simulink model "Motion_planner_Street_Drone"  (R2019b)
settings: Solver=FixedStepAuto  StartTime=0.0  StopTime=25  FixedStep=0.0075  MaxStep=1e-1  MinStep=1e-3  RelTol=1e-3  AbsTol=1e-4
InitFcn:
  | SD_init1
values from neighbouring files (symbols this model uses):
  cost = [2.71432892747 3.32441927977 3.79268757264 4.85642115368 6.12135035287 7.09825974303 9.57278659789 1.55754789407 1.51399555616 2.57723707661 3.8468529147 4.8336387623 ... (2430 elements, 1x2430)]    [matlab.mat]
  Front_brake = [0 2.2085352751 4.15209150797 6.12733711785 8.16604105928 9.79119154879 12.1808659635 14.1242630413 16.1155522836 18.1386900579 20.0839213981 22.1313006548 ... (68 elements, 34x2)]    [Front_brake.mat]
  N = size(X,1)    [curvature.m]
  obsx = [dx1 dx2 dx3 dx4]'    [dynamic_collison.m]    (also in dynamic_detection1.m = [x1 x2 x3 x4]')
  obsy = [dy1 dy2 dy3 dy4]'    [dynamic_collison.m]    (also in dynamic_detection1.m = [y1 y2 y3 y4]')
  x = obs_path(i,1)    [dynamic_collison.m]    (also in dynamic_detection1.m)
  X = [X]    [curvature.m]
  y = obs_path(i,2)    [dynamic_collison.m]    (also in dynamic_detection1.m)
undefined symbols (not defined in the file or in its folder): d, dfin, dini, Ki, Kp, L_0f, lookahead_time, lookahead_time_rev, Rear_brake, sigbuilder_block, steer_ratio, steer_sens, tfin, tini, TPS_0, xfin, Y, yfin, Z
libraries: sm_lib x290, nesl_utility x136, simulink x6, vrlib x2, powerlib_meascontrol x2
(part 2 of 14)

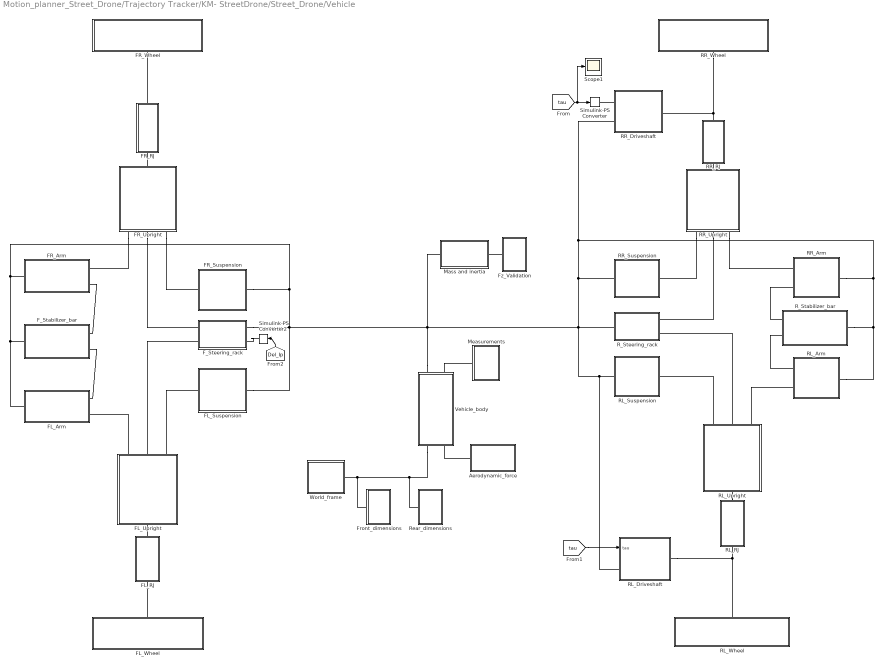
== system Motion_planner_Street_Drone/Trajectory Tracker/KM- StreetDrone/Street_Drone/Vehicle ==
  Aerodynamic_force : Subsystem
  FL_Arm : Subsystem
  FL_RJ : Subsystem
  FL_Suspension : Subsystem
  FL_Upright : Subsystem
  FL_Wheel : Subsystem
  FR_Arm : Subsystem
  FR_RJ : Subsystem
  FR_Suspension : Subsystem
  FR_Upright : Subsystem
  FR_Wheel : Subsystem
  F_Stabilizer_bar : Subsystem
  F_Steering_rack : Subsystem
  Front_dimensions : Subsystem
  Fz_Validation : Subsystem
  Mass and inertia : Subsystem
  Measurements : Subsystem
  RL_Arm : Subsystem
  RL_Driveshaft : Subsystem
  RL_RJ : Subsystem
  RL_Suspension : Subsystem
  RL_Upright : Subsystem
  RL_Wheel : Subsystem
  RR_Arm : Subsystem
  RR_Driveshaft : Subsystem
  RR_RJ : Subsystem
  RR_Suspension : Subsystem
  RR_Upright : Subsystem
  RR_Wheel : Subsystem
  R_Stabilizer_bar : Subsystem
  R_Steering_rack : Subsystem
  Rear_dimensions : Subsystem
  Scope1 : Scope
  Simulink-PS Converter : nesl_utility/Simulink-PS Converter  PhysicalDomain=network_engine_domain  SubClassName=ps_input  LeftPortType=input  RightPortType=output  PseudoPeriodic=off  Frequencies=[]  NoiseDistribution=none  NoiseParameters=[]  Unit=1  AffineConversion=off  FilteringAndDerivatives=provide  SimscapeFilterOrder=1  InputFilterTimeConstant=0.001  UdotUserProvided=0
  Simulink-PS Converter2 : nesl_utility/Simulink-PS Converter  PhysicalDomain=network_engine_domain  SubClassName=ps_input  LeftPortType=input  RightPortType=output  PseudoPeriodic=off  Frequencies=[]  NoiseDistribution=none  NoiseParameters=[]  Unit=cm  AffineConversion=off  FilteringAndDerivatives=filter  SimscapeFilterOrder=2  InputFilterTimeConstant=0.001  UdotUserProvided=0
  Vehicle_body : Subsystem
  World_frame : Subsystem
  wires:
  [tau] -> RL_Driveshaft/1(tau)
  [Del_Ip] -> Simulink-PS Converter2/1
  [tau] -> Simulink-PS Converter/1, Scope1/1
  connections:
  Fz_Validation/LConn1 -- Mass and inertia/RConn1
  RR_RJ/RConn1 -- RR_Wheel/LConn1 -- RR_Driveshaft/RConn1
  RL_RJ/RConn1 -- RL_Wheel/LConn1 -- RL_Driveshaft/RConn1
  FL_Wheel/LConn1 -- FL_RJ/RConn1
  FR_RJ/RConn1 -- FR_Wheel/LConn1
  FR_Arm/RConn2 -- F_Stabilizer_bar/RConn1
  Aerodynamic_force/LConn1 -- Vehicle_body/RConn2
  FR_Upright/LConn1 -- FR_Arm/RConn1
  RR_Upright/RConn1 -- RR_RJ/LConn1
  RR_Driveshaft/LConn1 -- Simulink-PS Converter/RConn1
  RL_Upright/LConn1 -- RL_RJ/LConn1
  Measurements/RConn1 -- Vehicle_body/LConn2
  World_frame/RConn1 -- Front_dimensions/LConn1 -- Rear_dimensions/LConn1 -- Vehicle_body/RConn1
  FL_Upright/RConn1 -- FL_RJ/LConn1
  RL_Upright/RConn1 -- RL_Suspension/RConn1
  RR_Upright/LConn1 -- RR_Suspension/RConn1
  FR_Upright/LConn2 -- F_Steering_rack/RConn1
  RR_Upright/LConn3 -- RR_Arm/RConn1
  FR_RJ/LConn1 -- FR_Upright/RConn1
  FL_Upright/LConn2 -- F_Steering_rack/RConn2
  RL_Upright/RConn3 -- RL_Arm/RConn2
  RR_Upright/LConn2 -- R_Steering_rack/RConn1
  Vehicle_body/LConn1 -- RR_Suspension/LConn1 -- RR_Arm/LConn1 -- RL_Arm/LConn1 -- R_Stabilizer_bar/LConn1 -- RR_Driveshaft/LConn2 -- R_Steering_rack/LConn1 -- RL_Suspension/LConn1 -- RL_Driveshaft/LConn1 -- Mass and inertia/LConn1 -- FL_Suspension/LConn1 -- F_Steering_rack/LConn1 -- FR_Suspension/LConn1 -- FR_Arm/LConn1 -- F_Stabilizer_bar/LConn1 -- FL_Arm/LConn1
  FR_Upright/LConn3 -- FR_Suspension/RConn1
  RL_Upright/RConn2 -- R_Steering_rack/RConn2
  R_Stabilizer_bar/RConn1 -- RR_Arm/RConn2
  Simulink-PS Converter2/RConn1 -- F_Steering_rack/LConn2
  FL_Upright/LConn1 -- FL_Arm/RConn2
  F_Stabilizer_bar/RConn2 -- FL_Arm/RConn1
  FL_Upright/LConn3 -- FL_Suspension/RConn1
  RL_Arm/RConn1 -- R_Stabilizer_bar/RConn2

== system Motion_planner_Street_Drone/Trajectory Tracker/KM- StreetDrone/Street_Drone/Inputs/Del ==
  del : Inport
  Constant2 : Constant  Value=0
  Del : Subsystem  Tag=STV Subsys  LoadFcn=sigbuilder_block('load');  StartFcn=sigbuilder_block('start');  StopFcn=sigbuilder_block('stop');  ClipboardFcn=sigbuilder_block('clipboard');  mask(Sigbuilder block){tuvar=[0:10]}
      mask help: Simulink:masks:SigbuilderBlock_MD
      mask init:
      | if ~strcmp(get_param(bdroot(gcbh),'SimulationStatus'),'stopped') tuvar = sigbuilder_block('maskInit'); end
      settings: CopyFcn=sigbuilder_block('copy');  DeleteFcn=sigbuilder_block('delete');  ModelCloseFcn=sigbuilder_block('modelClose');  PreSaveFcn=sigbuilder_block('preSave');  PauseFcn=sigbuilder_block('pause');  ContinueFcn=sigbuilder_block('continue');  NameChangeFcn=sigbuilder_block('namechange');  OpenFcn=sigbuilder_block('open',[5.4 72.6 1141.2 513.6 ]);  CloseFcn=sigbuilder_block('close');
      mask Display: plot(0, 0, 100, 100,[2, 2, 32, 32, 2], [68, 8, 8, 68, 68],[32, 2], [38, 38], [32, 19, 2],[53, 60, 44], [32, 17, 17, 2],[16, 16, 31, 31]);txt = getActiveGroup(gcbh);text(2, 100, txt,'verticalAlignment', 'top');
  Manual Switch1 : ManualSwitch
  Manual Switch3 : ManualSwitch  CurrentSetting=0
  Radius_of_pinion_cms : Gain  Gain=0.56
  Scope : Scope
  To Workspace : ToWorkspace  VariableName=del_hand_wheel  SampleTime=-1
  steering_ratio : Gain  Gain=14.0166
  to_degrees : Gain  Gain=180/pi
  to_radians : Gain  Gain=pi/180
  tag scope: Del_Ip=global, Del_Ip_hand=global
  wires:
  Del/1(Signal 1) -> Manual Switch1/2
  steering_ratio/1 -> Manual Switch1/1
  to_degrees/1 -> steering_ratio/1
  del/1 -> to_degrees/1
  Manual Switch3/1 -> Scope/1, [Del_Ip]
  Manual Switch1/1 -> To Workspace/1, [Del_Ip_hand], Radius_of_pinion_cms/1
  to_radians/1 -> Manual Switch3/2
  Radius_of_pinion_cms/1 -> to_radians/1
  Constant2/1 -> Manual Switch3/1

== system Motion_planner_Street_Drone/Trajectory Tracker/KM- StreetDrone/Street_Drone/Inputs/Velocity ==
  Vel : Inport
  Manual Switch2 : ManualSwitch  CurrentSetting=0
  Normal_manoever : Subsystem
  tag scope: Inputs=global
  wires:
  Vel/1 -> Manual Switch2/2
  Manual Switch2/1 -> [Inputs]
  Normal_manoever/1(Out1) -> Manual Switch2/1

== system Motion_planner_Street_Drone/Trajectory Tracker/KM- StreetDrone/Street_Drone/Powertrain and Brake System1/Brake_system ==
  I/p : Inport
  Brake_pedal : Saturate  UpperLimit=0  LowerLimit=-100
  Front_brake : Lookup_n-D  NumberOfTableDimensions=1  BreakpointsForDimension1=[Front_brake(:,1)]  Table=[Front_brake(:,2)]  InternalRulePriority=Speed  RndMeth=Simplest  InputSameDT=on
  Gain1 : Gain  Gain=-1
  Gain11 : Gain  Gain=-1/100
  Gain2 : Gain  Gain=0.5
  Gain3 : Gain  Gain=0.5
  Max_Br_pr : Gain  Gain=71.7
  Rear_brake : Lookup_n-D  NumberOfTableDimensions=1  BreakpointsForDimension1=[Rear_brake(:,1)]  Table=[Rear_brake(:,2)]  InternalRulePriority=Speed  RndMeth=Simplest  InputSameDT=on
  Scope{25,28..29,31} (4 alike) : Scope
  To Workspace1 : ToWorkspace  VariableName=brake_pr  SampleTime=-1
  To Workspace2 : ToWorkspace  VariableName=brake_pedal  SampleTime=-1
  tag scope: brTau_F=global, brTau_R=global, br_pedal=global
  wires:
  Gain3/1 -> [brTau_R]
  Gain2/1 -> [brTau_F]
  Max_Br_pr/1 -> Front_brake/1, To Workspace1/1, Scope31/1, Rear_brake/1
  Rear_brake/1 -> Scope28/1, Gain3/1
  Front_brake/1 -> Scope25/1, Gain2/1
  Gain11/1 -> Gain1/1, Max_Br_pr/1
  Brake_pedal/1 -> Scope29/1, Gain11/1
  I/p/1 -> Brake_pedal/1
  Gain1/1 -> To Workspace2/1, [br_pedal]

== system Motion_planner_Street_Drone/Trajectory Tracker/KM- StreetDrone/Street_Drone/Powertrain and Brake System1/Driveline_viscous_losses ==
  Gain : Gain  Gain=-1
  Product : Product
  Scope : Scope
  Scope1 : Scope
  Switch : Switch
  Viscous_friction1 : Gain  Commented=on  Gain=2
  Viscous_friction2 : Gain  Gain=2.537
  O/p : Outport
  tag scope: PT_loss=global
  wires:
  [motor_tau] -> Switch/2
  Gain/1 -> Switch/3
  Switch/1 -> O/p/1, Scope/1
  Product/1 -> Switch/1, Gain/1
  [RL_Re] -> Product/2
  Viscous_friction2/1 -> Product/1, Scope1/1, [PT_loss]
  [Vel] -> Viscous_friction2/1

== system Motion_planner_Street_Drone/Trajectory Tracker/KM- StreetDrone/Street_Drone/Powertrain and Brake System1/Motor ==
  I/p2 : Inport
  I/p1 : Inport  Port=2
  % : Gain  Gain=1/100
  %1 : Gain  Gain=100
  2-D Lookup Table2 : Lookup_n-D  BreakpointsForDimension1=[0 0.1 0.2 0.3 0.4 0.5 0.6 0.7 0.8 0.9 1]  BreakpointsForDimension2=[TPS_0(:,1)]  Table=[-90.24,-90.26,-90.24,-90.22,-90.23,-86.63,-72.71,-56.25,-50.21,-44.59,-40.69,-37.61,-34.44,-31.97,-29.79,-27.98,-26.37,-24.7,-23.15,-22.11,-21.24,-20.43,-19.47,-18.66,-17.94,-17.25,-16.58,-15.87,-15.16,-14.33,-14.11,-14.27,-14.21,-13.57,-12.89,-12.82,-12.72,-12.45,-12.19,-11.94,-11.65,-11.38,-10.97,-10.65;-25.48,-25.71,-26.16,-26.77,-27.52,-28.39,-29.45,-30.61,-30.61,-30.63,-30.66,-30.57,-29.83,-28.1,-26.6,-25.1,-23.88,-22.46,-21.12,-19.91,-18.49,-17.4,-16.44,-15.32,-14.29,-13.12,-11.74,-10.25,-9.37,-8.72,-8.56,-8.89,-9.14,-8.69,-8.35,-8.5,-8.76,-8.73,-8.69,-8.74,-8.78,-8.93,-8.85,-8.81;-3.28,-3.05,-2.62,-2.39,-2.44,-2.48,-2.54,-2.68,-2.6,-2.61,-2.62,-2.68,-2.68,-2.82,-2.75,-2.82,-2.8,-2.89,-2.94,-2.63,-2.34,-2.19,-2.46,-2.64,-2.54,-2.48,-2.51,-2.49,-2.26,-2.06,-2.09,-2.06,-2.16,-2.2,-2.19,-2.17,-2.12,-2.11,-2.09,-2.23,-2.18,-2.22,-1.91,-1.71;1.59,1.32,0.82,0.49,0.72,0.7,0.69,0.55,0.55,0.52,0.54,0.5,0.5,0.39,0.41,0.36,0.38,0.23,0.01,0.14,0.44,0.56,0.42,0.38,0.4,0.46,0.52,0.71,0.75,0.99,0.75,0.46,0.17,0.45,0.71,0.69,0.65,0.71,0.82,0.8,0.7,0.73,0.91,0.92;5.53,5.09,4.45,4.29,4.5,4.55,4.53,4.39,4.32,4.22,4.1,4.06,4.01,3.82,3.78,3.79,3.8,3.5,3.19,3.26,3.52,3.61,3.6,3.59,3.55,3.57,3.62,3.78,3.97,3.97,3.63,3.07,2.54,3,3.46,3.3,3.14,3.1,3.27,3.29,3.3,3.06,2.88,2.84;11.33,11.26,11.2,11.21,10.97,10.69,10.7,10.72,10.6,10.38,10.35,10.42,10.44,10.4,10.37,10.44,10.42,10.2,9.95,9.89,9.91,10,10.21,10.45,10.54,10.47,10.24,10,9.95,9.95,9.53,8.87,8.33,8.47,8.53,8.42,8.17,7.92,7.49,6.94,6.33,5.85,5.3,4.85;19.11,19.06,18.77,18.67,18.7,18.8,18.81,18.68,18.55,18.37,18.27,18.37,18.48,18.55,18.66,18.83,18.83,18.34,17.79,17.71,17.81,17.64,17.34,17.04,16.9,16.68,15.98,15.04,14.42,13.6,13.18,13.07,12.52,11.53,10.55,9.6,8.86,8.15,7.54,6.96,6.32,5.82,5.24,4.81;28.1,27.9,27.6,27.49,27.67,27.85,27.84,27.8,27.76,27.77,27.76,27.84,28.04,28.6,28.91,28.63,28.44,27.35,26.18,25.07,23.8,22.59,21.41,20.1,18.89,17.45,16.55,15.16,14.38,13.65,13.21,13.12,12.81,11.71,10.47,9.58,8.86,8.18,7.49,6.88,6.29,5.83,5.28,4.83;38.54,38.36,38.01,37.97,37.85,37.92,38.01,37.99,38.11,38.21,38.5,38.77,38.13,36.15,34.04,31.71,29.64,28.1,26.66,25.34,23.91,22.61,21.39,19.98,18.93,17.7,16.64,15.08,14.25,13.64,13.12,13.07,12.71,11.68,10.8,9.77,9.04,8.19,7.49,6.92,6.31,5.83,5.31,4.83;48.94,48.7,48.33,48.29,48.4,48.63,48.94,49.25,48.39,47.53,45.18,42.6,39.77,37.17,34.71,32.24,30.04,28.31,26.94,25.48,23.97,22.66,21.47,20.21,18.88,17.9,16.58,15.05,14.15,13.52,13.13,13.14,12.85,11.73,10.81,9.85,8.99,8.18,7.54,6.97,6.28,5.79,5.32,4.87;63.83,63.82,63.58,63.85,64.53,63.91,59.28,54.29,52.51,49.2,46.19,43.52,40.41,37.58,35.15,32.9,30.85,29.41,28.22,26.87,25.46,24.15,22.97,21.67,20.45,19.12,17.73,16.37,15.59,15.04,14.59,14.63,14.39,13.51,12.63,11.73,11.04,10.31,9.81,9.23,8.67,8.26,7.72,7.31]  InternalRulePriority=Speed  RndMeth=Simplest  InputSameDT=on
  2-D Lookup Table5 : Lookup_n-D  BreakpointsForDimension1=[0.3 0.4 0.5 0.6 0.7 0.8 0.9 1]  BreakpointsForDimension2=[TPS_0(:,1)]  Table=[1.59,1.32,0.82,0.49,0.72,0.7,0.69,0.55,0.55,0.52,0.54,0.5,0.5,0.39,0.41,0.36,0.38,0.23,0.01,0.14,0.44,0.56,0.42,0.38,0.4,0.46,0.52,0.71,0.75,0.99,0.75,0.46,0.17,0.45,0.71,0.69,0.65,0.71,0.82,0.8,0.7,0.73,0.91,0.92;5.53,5.09,4.45,4.29,4.5,4.55,4.53,4.39,4.32,4.22,4.1,4.06,4.01,3.82,3.78,3.79,3.8,3.5,3.19,3.26,3.52,3.61,3.6,3.59,3.55,3.57,3.62,3.78,3.97,3.97,3.63,3.07,2.54,3,3.46,3.3,3.14,3.1,3.27,3.29,3.3,3.06,2.88,2.84;11.33,11.26,11.2,11.21,10.97,10.69,10.7,10.72,10.6,10.38,10.35,10.42,10.44,10.4,10.37,10.44,10.42,10.2,9.95,9.89,9.91,10,10.21,10.45,10.54,10.47,10.24,10,9.95,9.95,9.53,8.87,8.33,8.47,8.53,8.42,8.17,7.92,7.49,6.94,6.33,5.85,5.3,4.85;19.11,19.06,18.77,18.67,18.7,18.8,18.81,18.68,18.55,18.37,18.27,18.37,18.48,18.55,18.66,18.83,18.83,18.34,17.79,17.71,17.81,17.64,17.34,17.04,16.9,16.68,15.98,15.04,14.42,13.6,13.18,13.07,12.52,11.53,10.55,9.6,8.86,8.15,7.54,6.96,6.32,5.82,5.24,4.81;28.1,27.9,27.6,27.49,27.67,27.85,27.84,27.8,27.76,27.77,27.76,27.84,28.04,28.6,28.91,28.63,28.44,27.35,26.18,25.07,23.8,22.59,21.41,20.1,18.89,17.45,16.55,15.16,14.38,13.65,13.21,13.12,12.81,11.71,10.47,9.58,8.86,8.18,7.49,6.88,6.29,5.83,5.28,4.83;38.54,38.36,38.01,37.97,37.85,37.92,38.01,37.99,38.11,38.21,38.5,38.77,38.13,36.15,34.04,31.71,29.64,28.1,26.66,25.34,23.91,22.61,21.39,19.98,18.93,17.7,16.64,15.08,14.25,13.64,13.12,13.07,12.71,11.68,10.8,9.77,9.04,8.19,7.49,6.92,6.31,5.83,5.31,4.83;48.94,48.7,48.33,48.29,48.4,48.63,48.94,49.25,48.39,47.53,45.18,42.6,39.77,37.17,34.71,32.24,30.04,28.31,26.94,25.48,23.97,22.66,21.47,20.21,18.88,17.9,16.58,15.05,14.15,13.52,13.13,13.14,12.85,11.73,10.81,9.85,8.99,8.18,7.54,6.97,6.28,5.79,5.32,4.87;63.83,63.82,63.58,63.85,64.53,63.91,59.28,54.29,52.51,49.2,46.19,43.52,40.41,37.58,35.15,32.9,30.85,29.41,28.22,26.87,25.46,24.15,22.97,21.67,20.45,19.12,17.73,16.37,15.59,15.04,14.59,14.63,14.39,13.51,12.63,11.73,11.04,10.31,9.81,9.23,8.67,8.26,7.72,7.31]  InternalRulePriority=Speed  RndMeth=Simplest  InputSameDT=on
  Derivative : Derivative
  Motor_rpm : Subsystem
  Saturation : Saturate  UpperLimit=1  LowerLimit=0.19
  Scope{,2,14,16,26,30,32} (7 alike) : Scope
  Switch : Switch  Criteria=u2 ~= 0
  Throttle : Saturate  UpperLimit=100  LowerLimit=0
  To Workspace : ToWorkspace  VariableName=tau  SampleTime=-1
  To Workspace1 : ToWorkspace  VariableName=throttle  SampleTime=-1
  condition_for_regen : simulink/Logic and Bit Operations/Compare To Constant  relop=>=  const=1  OutDataTypeStr=boolean
  O/p : Outport
  tag scope: motor_tau=global
  wires:
  Throttle/1 -> %/1
  %1/1 -> Scope26/1, To Workspace1/1
  Derivative/1 -> Scope/1
  I/p1/1 -> Throttle/1
  Switch/1 -> O/p/1, Scope16/1, Derivative/1, To Workspace/1, [motor_tau]
  2-D Lookup Table2/1 -> Scope30/1, Switch/1
  Saturation/1 -> 2-D Lookup Table5/1
  condition_for_regen/1 -> Scope2/1, Switch/2
  2-D Lookup Table5/1 -> Scope14/1, Switch/3
  Motor_rpm/1(Out1) -> 2-D Lookup Table2/2, 2-D Lookup Table5/2
  %/1 -> %1/1, 2-D Lookup Table2/1, Saturation/1, Scope32/1
  I/p2/1 -> condition_for_regen/1

== system Motion_planner_Street_Drone/Trajectory Tracker/KM- StreetDrone/Street_Drone/Powertrain and Brake System1/Scaling ==
  I/p : Inport
  Constant : Constant  Value=112.3
  Motor_gain : Gain  Gain=1.086
  Product : Product
  Scope : Scope
  Scope1 : Scope
  Subtract2 : Sum
  O/p : Outport
  tag scope: Before_gear=global
  wires:
  Product/1 -> Scope/1, Subtract2/2
  [RL_Re] -> Product/2
  Constant/1 -> Product/1
  I/p/1 -> Motor_gain/1
  Subtract2/1 -> O/p/1, [Before_gear]
  Motor_gain/1 -> Subtract2/1, Scope1/1

== system Motion_planner_Street_Drone/Trajectory Tracker/KM- StreetDrone/Street_Drone/Results1/Actual brake torque ==
  Add : Sum
  Add1 : Sum
  Scope : Scope  NumInputPorts=2
  Scope1 : Scope
  Scope2 : Scope  NumInputPorts=2
  Scope3 : Scope
  To Workspace : ToWorkspace  VariableName=brTau_F  SampleTime=-1
  To Workspace2 : ToWorkspace  VariableName=brTau_R  SampleTime=-1
  wires:
  Add1/1 -> Scope3/1, To Workspace2/1
  [act_br_RL] -> Scope2/1, Add1/1
  [act_br_RR] -> Add1/2, Scope2/2
  [act_br_FR] -> Scope/2, Add/2
  [act_br_FL] -> Add/1, Scope/1
  Add/1 -> To Workspace/1, Scope1/1

== system Motion_planner_Street_Drone/Trajectory Tracker/KM- StreetDrone/Street_Drone/Results1/Ay&Yaw ==
  Divide4 : Product  Inputs=*/
  Scope1 : Scope
  Scope14 : Scope
  To Workspace1 : ToWorkspace  VariableName=Yaw  SampleTime=-1
  To Workspace4 : ToWorkspace  VariableName=ay  SampleTime=-1
  wires:
  [Yaw_rate] -> Scope1/1, To Workspace1/1
  [mass] -> Divide4/2
  Divide4/1 -> To Workspace4/1, Scope14/1
  [Fy_total] -> Divide4/1

== system Motion_planner_Street_Drone/Trajectory Tracker/KM- StreetDrone/Street_Drone/Results1/Coordinates ==
  Scope12 : Scope
  Scope16 : Scope
  To Workspace2 : ToWorkspace  VariableName=Y_SD  SampleTime=-1
  To Workspace8 : ToWorkspace  VariableName=X_SD  SampleTime=-1
  wires:
  [Y] -> To Workspace2/1, Scope16/1
  [X] -> To Workspace8/1, Scope12/1

== system Motion_planner_Street_Drone/Trajectory Tracker/KM- StreetDrone/Street_Drone/Results1/Fx ==
  Actual : Subsystem
  Calculated : Subsystem

== system Motion_planner_Street_Drone/Trajectory Tracker/KM- StreetDrone/Street_Drone/Results1/Fy ==
  Add3 : Sum  Inputs=++++
  Add4 : Sum
  Add5 : Sum
  Gain3 : Gain  Gain=-1
  Scope24 : Scope
  Scope31 : Scope  NumInputPorts=2
  Scope32 : Scope  NumInputPorts=2
  Scope4 : Scope
  Scope5 : Scope
  To Workspace : ToWorkspace  VariableName=Fy_front  SampleTime=-1
  To Workspace1 : ToWorkspace  VariableName=Fy_rear  SampleTime=-1
  To Workspace10 : ToWorkspace  VariableName=actual_Fy_vehicle  SampleTime=-1
  To Workspace11 : ToWorkspace  VariableName=actual_Fy_RL  SampleTime=-1
  To Workspace12 : ToWorkspace  VariableName=actual_Fy_RR  SampleTime=-1
  tag scope: Fy_F=global, Fy_R=global, Fy_total=global
  wires:
  [FL_Fy] -> Add4/1, Add3/1, Scope31/1
  [RL_Fy] -> Add3/3, Scope32/1, To Workspace11/1, Add5/1
  Gain3/1 -> Add3/4, Add5/2, To Workspace12/1, Scope32/2
  [RR_Fy] -> Gain3/1
  [FR_Fy] -> Add3/2, Scope31/2, Add4/2
  Add3/1 -> [Fy_total], To Workspace10/1, Scope24/1
  Add4/1 -> To Workspace/1, [Fy_F], Scope4/1
  Add5/1 -> To Workspace1/1, Scope5/1, [Fy_R]

== system Motion_planner_Street_Drone/Trajectory Tracker/KM- StreetDrone/Street_Drone/Results1/Fz ==
  Plot Tire Results : Subsystem
      settings: OpenFcn=PlotTireOutputs_UI
      mask Display: disp('Plot Tire Results');
  Sensing : Subsystem
  Tire Forces : Scope
  wires:
  Sensing/1(Fz) -> Tire Forces/1

== system Motion_planner_Street_Drone/Trajectory Tracker/KM- StreetDrone/Street_Drone/Results1/Steering_angle ==
  Constant : Constant  Value=0.01683
  Gain : Gain  Gain=0.5
  Gain1 : Gain  Gain=180/pi
  Gain2 : Gain  Gain=180/pi
  Gain3 : Gain  Gain=180/pi
  Scope{,1..2,7} (4 alike) : Scope
  Subtract : Sum  Inputs=+-
  Subtract1 : Sum
  Subtract2 : Sum
  To Workspace1 : ToWorkspace  VariableName=del_road_wheel  SampleTime=-1
  To Workspace15 : ToWorkspace  VariableName=Del  SampleTime=-1
  To Workspace2 : ToWorkspace  VariableName=del_road_wheel_L  SampleTime=-1
  To Workspace3 : ToWorkspace  VariableName=del_road_wheel_R  SampleTime=-1
  actual_wheel_steering_angle : Display
  tag scope: Del_Act_Ang=global, Del_Op=global
  wires:
  Gain3/1 -> To Workspace3/1
  Gain2/1 -> To Workspace2/1
  Gain/1 -> Gain1/1, [Del_Op], To Workspace15/1, Scope7/1
  [Del_L] -> Subtract/1
  Subtract1/1 -> Scope/1, Gain3/1, Subtract2/2
  [Del_R] -> Subtract1/2
  Subtract/1 -> Scope1/1, Gain2/1, Subtract2/1
  Constant/1 -> Subtract1/1, Subtract/2
  Subtract2/1 -> Gain/1
  Gain1/1 -> Scope2/1, [Del_Act_Ang], To Workspace1/1, actual_wheel_steering_angle/1

== system Motion_planner_Street_Drone/Trajectory Tracker/KM- StreetDrone/Street_Drone/Results1/Subsystem1 ==
  Add : Sum
  Add1 : Sum  Inputs=++++
  Add2 : Sum
  Gain : Gain  Gain=0.0151
  Scope{,1..4} (5 alike) : Scope
  To Workspace : ToWorkspace  VariableName=Drag_force  SampleTime=-1
  To Workspace1 : ToWorkspace  VariableName=Total_long_force  SampleTime=-1
  tag scope: Drag_force=global, Total_long_force=global
  wires:
  Gain/1 -> Add1/3, Scope2/1
  Add2/1 -> Scope1/1, To Workspace1/1, [Total_long_force]
  [Fx] -> Add2/2, Scope4/1
  Add1/1 -> Scope/1, Add2/1, [Drag_force], To Workspace/1
  Add/1 -> Add1/4, Scope3/1
  [Iner_loss_R] -> Add/2
  [Iner_loss_L] -> Add/1
  [Fz_total] -> Gain/1
  [PT_loss] -> Add1/1
  [Aero_loss] -> Add1/2

== system Motion_planner_Street_Drone/Trajectory Tracker/KM- StreetDrone/Street_Drone/Results1/Velocity&Ax ==
  Add1 : Sum  Inputs=++++
  Derivative : Derivative
  Display : Display
  Gain : Gain  Gain=-1
  Gain1 : Gain  Gain=3.6
  Gain9 : Gain  Gain=0.25
  Saturation : Saturate  UpperLimit=25  LowerLimit=0
  Scope : Scope
  Scope1 : Scope
  Scope2 : Scope
  Scope3 : Scope  NumInputPorts=4
  To Workspace1 : ToWorkspace  VariableName=Actual_Vel  SampleTime=-1
  To Workspace2 : ToWorkspace  VariableName=Act_Ax  SampleTime=-1
  tag scope: Act_Ax=global, Vel=global
  wires:
  Gain9/1 -> Derivative/1, Saturation/1, [Vel], Scope/1, Gain1/1, Display/1
  Gain1/1 -> Scope2/1
  Derivative/1 -> [Act_Ax], To Workspace2/1, Scope1/1
  [FL_Vx] -> Add1/1, Scope3/1
  [RR_Vx] -> Gain/1
  [RL_Vx] -> Add1/3, Scope3/3
  [FR_Vx] -> Add1/2, Scope3/2
  Gain/1 -> Add1/4, Scope3/4
  Add1/1 -> Gain9/1
  Saturation/1 -> To Workspace1/1

== system Motion_planner_Street_Drone/Trajectory Tracker/KM- StreetDrone/Street_Drone/Vehicle/Aerodynamic_force ==
  External Force and Torque : sm_lib/Forces and Torques/External Force and Torque  ForceResolutionFrame=AttachedFrame  EnableForceX=on  EnableForceY=off  EnableForceZ=off  EnableForce=off  TorqueResolutionFrame=AttachedFrame  EnableTorqueX=off  EnableTorqueY=off  EnableTorqueZ=off  EnableTorque=off
  Gain : Gain  Gain=0.5
  Product : Product  Inputs=3
  Rigid Transform : sm_lib/Frames and Transforms/Rigid Transform  TranslationMethod=Cartesian  TranslationStandardOffset=1.169  TranslationLengthUnit=m  TranslationStandardAxis=+X  TranslationCartesianOffset=[1.169 0 -0.1305]  TranslationROffset=0  TranslationROffsetUnits=m  TranslationZOffset=0  TranslationZOffsetUnits=m  TranslationThetaOffset=0  TranslationThetaOffsetUnits=deg  RotationMethod=StandardAxis  RotationAngleUnits=deg  RotationStandardAxis=+Z  RotationAngle=180  RotationArbitraryAxis=[0 0 1]  FollAlignAxisA=+X  BaseAlignAxisA=+Y  FollAlignAxisB=+Y  BaseAlignAxisB=+Z  RotationSequenceAxes=FollowerAxes  RotationSequence=XYX  RotationSequenceAngles=[0 0 0]  RotationSequenceAnglesUnits=deg  RotationMatrix=[1 0 0; 0 1 0; 0 0 1]
  Scope : Scope
  Simulink-PS Converter3 : nesl_utility/Simulink-PS Converter  PhysicalDomain=network_engine_domain  SubClassName=ps_input  LeftPortType=input  RightPortType=output  PseudoPeriodic=off  Frequencies=[]  NoiseDistribution=none  NoiseParameters=[]  Unit=1  AffineConversion=off  FilteringAndDerivatives=provide  SimscapeFilterOrder=1  InputFilterTimeConstant=0.001  UdotUserProvided=0
  row*SCx : Constant  Value=0.81
  row*SCx1 : Constant  Value=0.804288
  vehicle_body : PMIOPort  Side=Left
  tag scope: Aero_loss=global
  wires:
  Product/1 -> Gain/1
  [Vel] -> Product/2
  [Vel] -> Product/3
  Gain/1 -> Simulink-PS Converter3/1, Scope/1, [Aero_loss]
  row*SCx1/1 -> Product/1
  connections:
  Rigid Transform/RConn1 -- External Force and Torque/RConn1
  Simulink-PS Converter3/RConn1 -- External Force and Torque/LConn1
  Rigid Transform/LConn1 -- vehicle_body/RConn1

== system Motion_planner_Street_Drone/Trajectory Tracker/KM- StreetDrone/Street_Drone/Vehicle/FL_Arm ==
  FL arm : sm_lib/Body Elements/Extruded Solid  GraphicAmbientColor=[0.15 0.15 0.15 1.0]  BasedOnType=Mass  CenterOfMass=[0 0 0]  CenterOfMassUnits=m  GraphicDiffuseColor=[0.5 0.5 0.5]  ExtrusionCrossSection=[10 14.471; -10 14.471; -10 -14.471; 10 -14.471]  ExtrusionCrossSectionUnits=cm  Density=1000  DensityUnits=kg/m^3  DoExposeReferenceFrame=off  GraphicEmissiveColor=[0.0 0.0 0.0 1.0]  ExportEntireGeometry=off  ExtrusionLength=1  ExtrusionLengthUnits=cm  ExtrusionType=General  SerializedFrames=<Frames><Frame><Id>Frame1</Id><Value><Name>F1</Name><Origin><Source>GeometricFeature</Source><FeatureName>side surface 3</FeatureName></Origin><PrimaryAxis><DefinedDirection>+X</DefinedDirection><Source>ReferenceFrame</Source><SourceDirection>+Z</SourceDirection><FeatureName></FeatureName></PrimaryAxis><SecondaryAxis><DefinedDirection>+Y</DefinedDirection><Source>ReferenceFrame</Source><SourceDirection>+Y</SourceDirection><FeatureName></FeatureName></SecondaryAxis></Value></Frame><Frame><Id>Frame2</Id><Value><Name>F2</Name><Origin><Source>GeometricFeature</Source><FeatureName>side surface 1</FeatureName></Origin><PrimaryAxis><DefinedDirection>+Z</DefinedDirection><Source>ReferenceFrame</Source><SourceDirection>+Y</SourceDirection><FeatureName></FeatureName></PrimaryAxis><SecondaryAxis><DefinedDirection>+Y</DefinedDirection><Source>ReferenceFrame</Source><SourceDirection>+X</SourceDirection><FeatureName></FeatureName></SecondaryAxis></Value></Frame></Frames>  MarkerShape=Sphere  MarkerSize=10  GraphicType=FromGeometry  InertiaType=CalculateFromGeometry  Mass=3  MassUnits=kg  MomentsOfInertia=[1 1 1]  MomentsOfInertiaUnits=kg*m^2  PolygonNumSides=3  GraphicOpacity=1.0  PolygonOuterRadius=1  PolygonOuterRadiusUnits=m  ProductsOfInertia=[0 0 0]  ProductsOfInertiaUnits=kg*m^2  GraphicShininess=75  GraphicSpecularColor=[0.5 0.5 0.5 1.0]  GraphicVisPropType=SimpleVisualProperties
  Revolute Joint : sm_lib/Joints/Revolute Joint  JointMode=Normal  SenseConstraintForce=off  SenseConstraintForceX=off  SenseConstraintForceY=off  SenseConstraintForceZ=off  SenseConstraintTorque=off  SenseConstraintTorqueX=off  SenseConstraintTorqueY=off  SenseConstraintTorqueZ=off  SenseTotalForce=off  SenseTotalForceX=off  SenseTotalForceY=off  SenseTotalForceZ=off  SenseTotalTorque=off  SenseTotalTorqueX=off  SenseTotalTorqueY=off  SenseTotalTorqueZ=off  CompositeWrenchDir=FollowerOnBase  CompositeWrenchFrame=BaseFrame  EquilibriumPosition=0  EquilibriumPositionUnits=deg  SpringStiffness=0  SpringStiffnessUnits=N*m/deg  DampingCoefficient=0  DampingCoefficientUnits=N*m/(deg/s)  TorqueActuationMode=NoTorque  MotionActuationMode=ComputedMotion  SensePosition=off  SenseVelocity=off  SenseAcceleration=off  SenseTorqueForce=off  SenseLowerLimitTorqueForce=off  SenseUpperLimitTorqueForce=off  LowerLimitSpecify=off  LowerLimitBound=-90  LowerLimitBoundUnits=deg  LowerLimitStiffness=1e4  LowerLimitStiffnessUnits=N*m/deg  LowerLimitDamping=10  LowerLimitDampingUnits=N*m/(deg/s)  LowerLimitTransitionRegionWidth=0.1  LowerLimitTransitionRegionWidthUnits=deg  UpperLimitSpecify=off  UpperLimitBound=90  UpperLimitBoundUnits=deg  UpperLimitStiffness=1e4  UpperLimitStiffnessUnits=N*m/deg  UpperLimitDamping=10  UpperLimitDampingUnits=N*m/(deg/s)  UpperLimitTransitionRegionWidth=0.1  UpperLimitTransitionRegionWidthUnits=deg  PositionTargetSpecify=off  PositionTargetPriority=High  PositionTargetValue=0  PositionTargetValueUnits=deg  VelocityTargetSpecify=off  VelocityTargetPriority=High  VelocityTargetValue=0  VelocityTargetValueUnits=deg/s
  Rigid Transform1 : sm_lib/Frames and Transforms/Rigid Transform  TranslationMethod=Cartesian  TranslationStandardOffset=0  TranslationLengthUnit=m  TranslationStandardAxis=+Z  TranslationCartesianOffset=[0.03625 -0.08055 -0.0027]  TranslationROffset=0  TranslationROffsetUnits=m  TranslationZOffset=0  TranslationZOffsetUnits=m  TranslationThetaOffset=0  TranslationThetaOffsetUnits=deg  RotationMethod=None  RotationAngleUnits=deg  RotationStandardAxis=+Z  RotationAngle=0.0  RotationArbitraryAxis=[0 0 1]  FollAlignAxisA=+X  BaseAlignAxisA=-Y  FollAlignAxisB=+Y  BaseAlignAxisB=+Z  RotationSequenceAxes=FollowerAxes  RotationSequence=XYX  RotationSequenceAngles=[0 0 0]  RotationSequenceAnglesUnits=deg  RotationMatrix=[1 0 0; 0 1 0; 0 0 1]
  Rigid Transform13 : sm_lib/Frames and Transforms/Rigid Transform  TranslationMethod=None  TranslationStandardOffset=0  TranslationLengthUnit=m  TranslationStandardAxis=+Z  TranslationCartesianOffset=[0.0377 0.08337 -0.1277]  TranslationROffset=0  TranslationROffsetUnits=m  TranslationZOffset=0  TranslationZOffsetUnits=m  TranslationThetaOffset=0  TranslationThetaOffsetUnits=deg  RotationMethod=AlignedAxes  RotationAngleUnits=deg  RotationStandardAxis=+Z  RotationAngle=0.0  RotationArbitraryAxis=[0 0 1]  FollAlignAxisA=+X  BaseAlignAxisA=-Y  FollAlignAxisB=+Y  BaseAlignAxisB=+Z  RotationSequenceAxes=FollowerAxes  RotationSequence=XYX  RotationSequenceAngles=[0 0 0]  RotationSequenceAnglesUnits=deg  RotationMatrix=[1 0 0; 0 1 0; 0 0 1]
  Rigid Transform7 : sm_lib/Frames and Transforms/Rigid Transform  TranslationMethod=Cartesian  TranslationStandardOffset=0  TranslationLengthUnit=m  TranslationStandardAxis=+Z  TranslationCartesianOffset=[0.97281 0.17335 -0.27437]  TranslationROffset=0  TranslationROffsetUnits=m  TranslationZOffset=0  TranslationZOffsetUnits=m  TranslationThetaOffset=0  TranslationThetaOffsetUnits=deg  RotationMethod=None  RotationAngleUnits=deg  RotationStandardAxis=+Z  RotationAngle=0.0  RotationArbitraryAxis=[0 0 1]  FollAlignAxisA=+X  BaseAlignAxisA=+Y  FollAlignAxisB=+Y  BaseAlignAxisB=+Z  RotationSequenceAxes=FollowerAxes  RotationSequence=XYX  RotationSequenceAngles=[0 0 0]  RotationSequenceAnglesUnits=deg  RotationMatrix=[1 0 0; 0 1 0; 0 0 1]
  Rigid Transform8 : sm_lib/Frames and Transforms/Rigid Transform  TranslationMethod=None  TranslationStandardOffset=0  TranslationLengthUnit=m  TranslationStandardAxis=+Z  TranslationCartesianOffset=[0.9728 0.173 -0.274]  TranslationROffset=0  TranslationROffsetUnits=m  TranslationZOffset=0  TranslationZOffsetUnits=m  TranslationThetaOffset=0  TranslationThetaOffsetUnits=deg  RotationMethod=StandardAxis  RotationAngleUnits=deg  RotationStandardAxis=+Y  RotationAngle=90  RotationArbitraryAxis=[0 0 1]  FollAlignAxisA=+X  BaseAlignAxisA=+Y  FollAlignAxisB=+Y  BaseAlignAxisB=+Z  RotationSequenceAxes=FollowerAxes  RotationSequence=XYX  RotationSequenceAngles=[0 0 0]  RotationSequenceAnglesUnits=deg  RotationMatrix=[1 0 0; 0 1 0; 0 0 1]
  Spherical Joint1 : sm_lib/Joints/Spherical Joint  JointMode=Normal  SenseConstraintForce=off  SenseConstraintForceX=off  SenseConstraintForceY=off  SenseConstraintForceZ=off  SenseConstraintTorque=off  SenseConstraintTorqueX=off  SenseConstraintTorqueY=off  SenseConstraintTorqueZ=off  SenseTotalForce=off  SenseTotalForceX=off  SenseTotalForceY=off  SenseTotalForceZ=off  SenseTotalTorque=off  SenseTotalTorqueX=off  SenseTotalTorqueY=off  SenseTotalTorqueZ=off  CompositeWrenchDir=FollowerOnBase  CompositeWrenchFrame=BaseFrame  DefPosRotationMethod=None  DefPosRotationAngleUnits=deg  DefPosRotationStandardAxis=+Z  DefPosRotationAngle=0.0  DefPosRotationArbitraryAxis=[0 0 1]  DefPosFollAlignAxisA=+X  DefPosBaseAlignAxisA=+Y  DefPosFollAlignAxisB=+Y  DefPosBaseAlignAxisB=+Z  DefPosRotationSequenceAxes=FollowerAxes  DefPosRotationSequence=XYX  DefPosRotationSequenceAngles=[0 0 0]  DefPosRotationSequenceAnglesUnits=deg  DefPosRotationMatrix=[1 0 0; 0 1 0; 0 0 1]  EqPosRotationMethod=None  EqPosRotationAngleUnits=deg  EqPosRotationStandardAxis=+Z  EqPosRotationAngle=0.0  EqPosRotationArbitraryAxis=[0 0 1]  EqPosFollAlignAxisA=+X  EqPosBaseAlignAxisA=+Y  EqPosFollAlignAxisB=+Y  EqPosBaseAlignAxisB=+Z  EqPosRotationSequenceAxes=FollowerAxes  EqPosRotationSequence=XYX  EqPosRotationSequenceAngles=[0 0 0]  EqPosRotationSequenceAnglesUnits=deg  EqPosRotationMatrix=[1 0 0; 0 1 0; 0 0 1]  SpringStiffness=0  SpringStiffnessUnits=N*m/deg  DampingCoefficient=0  DampingCoefficientUnits=N*m/(deg/s)  ActuateTorqueX=on  ActuateTorqueY=on  ActuateTorqueZ=on  ActuateTorque=off  TorqueActuationMode=NoTorque  MotionActuationMode=ComputedMotion  ActuationFrame=BaseFrame  SensePosition=off  SenseVelocityX=off  SenseVelocityY=off  SenseVelocityZ=off  SenseVelocity=off  SenseAccelerationX=off  SenseAccelerationY=off  SenseAccelerationZ=off  SenseAcceleration=off  SenseTorqueX=off  SenseTorqueY=off  SenseTorqueZ=off  SenseTorqueForce=off  SenseLowerLimitTorqueMag=off  SenseUpperLimitTorqueMag=off  SensingFrame=BaseFrame  LowerLimitSpecify=off  LowerLimitBound=15  LowerLimitBoundUnits=deg  LowerLimitStiffness=1e4  LowerLimitStiffnessUnits=N*m/deg  LowerLimitDamping=10  LowerLimitDampingUnits=N*m/(deg/s)  LowerLimitTransitionRegionWidth=0.1  LowerLimitTransitionRegionWidthUnits=deg  UpperLimitSpecify=off  UpperLimitBound=45  UpperLimitBoundUnits=deg  UpperLimitStiffness=1e4  UpperLimitStiffnessUnits=N*m/deg  UpperLimitDamping=10  UpperLimitDampingUnits=N*m/(deg/s)  UpperLimitTransitionRegionWidth=0.1  UpperLimitTransitionRegionWidthUnits=deg  PositionTargetRotationMethod=None  PositionTargetRotationAngleUnits=deg  PositionTargetRotationStandardAxis=+Z  PositionTargetRotationAngle=0.0  PositionTargetRotationArbitraryAxis=[0 0 1]  PositionTargetFollAlignAxisA=+X  PositionTargetBaseAlignAxisA=+Y  PositionTargetFollAlignAxisB=+Y  PositionTargetBaseAlignAxisB=+Z  PositionTargetRotationSequenceAxes=FollowerAxes  PositionTargetRotationSequence=XYX  PositionTargetRotationSequenceAngles=[0 0 0]  PositionTargetRotationSequenceAnglesUnits=deg  PositionTargetRotationMatrix=[1 0 0; 0 1 0; 0 0 1]  PositionTargetSpecify=off  PositionTargetPriority=High  VelocityTargetValue=[0 0 0]  VelocityTargetValueUnits=deg/s  VelocityTargetSpecify=off  VelocityTargetPriority=Low  VelocityTargetInFollowerFrame=off
  chassis : PMIOPort  Side=Left
  stabilizer_bar : PMIOPort  Port=2  Side=Right
  upright : PMIOPort  Port=3  Side=Right
  connections:
  Rigid Transform1/RConn1 -- stabilizer_bar/RConn1
  upright/RConn1 -- Spherical Joint1/RConn1
  Rigid Transform7/LConn1 -- chassis/RConn1
  Spherical Joint1/LConn1 -- Rigid Transform1/LConn1 -- Rigid Transform13/RConn1
  Rigid Transform8/LConn1 -- Rigid Transform7/RConn1
  Rigid Transform8/RConn1 -- Revolute Joint/LConn1
  FL arm/LConn1 -- Revolute Joint/RConn1
  FL arm/RConn1 -- Rigid Transform13/LConn1

== system Motion_planner_Street_Drone/Trajectory Tracker/KM- StreetDrone/Street_Drone/Vehicle/FL_RJ ==
  Gain : Gain  Gain=-1
  PS-Simulink Converter : nesl_utility/PS-Simulink Converter  PhysicalDomain=network_engine_domain  SubClassName=ps_output  LeftPortType=input  RightPortType=output  PseudoPeriodic=off  Frequencies=[]  Unit=inherit  AffineConversion=off
  PS-Simulink Converter1 : nesl_utility/PS-Simulink Converter  PhysicalDomain=network_engine_domain  SubClassName=ps_output  LeftPortType=input  RightPortType=output  PseudoPeriodic=off  Frequencies=[]  Unit=inherit  AffineConversion=off
  PS-Simulink Converter2 : nesl_utility/PS-Simulink Converter  PhysicalDomain=network_engine_domain  SubClassName=ps_output  LeftPortType=input  RightPortType=output  PseudoPeriodic=off  Frequencies=[]  Unit=inherit  AffineConversion=off
  RJ_FL : sm_lib/Joints/Revolute Joint  JointMode=Normal  SenseConstraintForce=off  SenseConstraintForceX=off  SenseConstraintForceY=off  SenseConstraintForceZ=off  SenseConstraintTorque=off  SenseConstraintTorqueX=off  SenseConstraintTorqueY=off  SenseConstraintTorqueZ=off  SenseTotalForce=off  SenseTotalForceX=off  SenseTotalForceY=off  SenseTotalForceZ=off  SenseTotalTorque=off  SenseTotalTorqueX=off  SenseTotalTorqueY=off  SenseTotalTorqueZ=off  CompositeWrenchDir=FollowerOnBase  CompositeWrenchFrame=BaseFrame  EquilibriumPosition=0  EquilibriumPositionUnits=deg  SpringStiffness=0  SpringStiffnessUnits=N*m/deg  DampingCoefficient=0  DampingCoefficientUnits=N*m/(deg/s)  TorqueActuationMode=InputTorque  MotionActuationMode=ComputedMotion  SensePosition=off  SenseVelocity=on  SenseAcceleration=on  SenseTorqueForce=on  SenseLowerLimitTorqueForce=off  SenseUpperLimitTorqueForce=off  LowerLimitSpecify=off  LowerLimitBound=-90  LowerLimitBoundUnits=deg  LowerLimitStiffness=1e4  LowerLimitStiffnessUnits=N*m/deg  LowerLimitDamping=10  LowerLimitDampingUnits=N*m/(deg/s)  LowerLimitTransitionRegionWidth=0.1  LowerLimitTransitionRegionWidthUnits=deg  UpperLimitSpecify=off  UpperLimitBound=90  UpperLimitBoundUnits=deg  UpperLimitStiffness=1e4  UpperLimitStiffnessUnits=N*m/deg  UpperLimitDamping=10  UpperLimitDampingUnits=N*m/(deg/s)  UpperLimitTransitionRegionWidth=0.1  UpperLimitTransitionRegionWidthUnits=deg  PositionTargetSpecify=off  PositionTargetPriority=High  PositionTargetValue=0  PositionTargetValueUnits=deg  VelocityTargetSpecify=off  VelocityTargetPriority=High  VelocityTargetValue=52.39  VelocityTargetValueUnits=rad/s
  Rigid Transform2 : sm_lib/Frames and Transforms/Rigid Transform  TranslationMethod=StandardAxis  TranslationStandardOffset=4  TranslationLengthUnit=cm  TranslationStandardAxis=+Z  TranslationCartesianOffset=[0 0 0]  TranslationROffset=0  TranslationROffsetUnits=m  TranslationZOffset=0  TranslationZOffsetUnits=m  TranslationThetaOffset=0  TranslationThetaOffsetUnits=deg  RotationMethod=None  RotationAngleUnits=deg  RotationStandardAxis=+Z  RotationAngle=0.0  RotationArbitraryAxis=[0 0 1]  FollAlignAxisA=+X  BaseAlignAxisA=+Y  FollAlignAxisB=+Y  BaseAlignAxisB=+Z  RotationSequenceAxes=FollowerAxes  RotationSequence=XYX  RotationSequenceAngles=[0 0 0]  RotationSequenceAnglesUnits=deg  RotationMatrix=[1 0 0; 0 1 0; 0 0 1]
  Scope : Scope  NumInputPorts=3
  Scope1 : Scope
  Simulink-PS Converter : nesl_utility/Simulink-PS Converter  PhysicalDomain=network_engine_domain  SubClassName=ps_input  LeftPortType=input  RightPortType=output  PseudoPeriodic=off  Frequencies=[]  NoiseDistribution=none  NoiseParameters=[]  Unit=1  AffineConversion=off  FilteringAndDerivatives=provide  SimscapeFilterOrder=1  InputFilterTimeConstant=0.001  UdotUserProvided=0
  Switch : Switch  Criteria=u2 > Threshold
  upright : PMIOPort  Side=Left
  wheel : PMIOPort  Port=2  Side=Right
  tag scope: act_br_FL=global
  wires:
  [brTau_F] -> Switch/1, Gain/1
  [Vel] -> Switch/2
  Gain/1 -> Switch/3
  Switch/1 -> Simulink-PS Converter/1, Scope1/1
  PS-Simulink Converter2/1 -> Scope/3, [act_br_FL]
  PS-Simulink Converter1/1 -> Scope/2
  PS-Simulink Converter/1 -> Scope/1
  connections:
  Rigid Transform2/RConn1 -- RJ_FL/RConn1
  Simulink-PS Converter/RConn1 -- RJ_FL/LConn2
  PS-Simulink Converter2/LConn1 -- RJ_FL/RConn4
  PS-Simulink Converter1/LConn1 -- RJ_FL/RConn3
  PS-Simulink Converter/LConn1 -- RJ_FL/RConn2
  RJ_FL/LConn1 -- upright/RConn1
  wheel/RConn1 -- Rigid Transform2/LConn1
